simulink model "sim_process_power_old"  (Simulink 9.3)
settings: Solver=VariableStepAuto  StartTime=0.0  StopTime=0.1  MaxStep=1/25e3  RelTol=1e-3
settings Model: Creator=VMORAIS  LastModifiedBy=VMORAIS
settings DataIOCC: SaveFormat=Dataset  SignalLoggingSaveFormat=Dataset  ReturnWorkspaceOutputs=on
settings OptimizationCC: LifeSpan=auto
settings DebuggingCC: UnderspecifiedInitializationDetection=Simplified  MergeDetectMultiDrivingBlocksExec=error  FcnCallInpInsideContextMsg=error  SFUnexpectedBacktrackingDiag=error  SFNoUnconditionalDefaultTransitionDiag=error  SFExecutionAtInitializationDiag=warning  SFMachineParentedDataDiag=error  ArithmeticOperatorsInVariantConditions=error
settings HardwareCC: ProdBitPerPointer=64  ProdBitPerSizeT=64  ProdBitPerPtrDiffT=64  ProdLargestAtomicFloat=Float  ProdIntDivRoundTo=Zero  ProdEndianess=LittleEndian  ProdWordSize=64  ProdHWDeviceType=Intel->x86-64 (Windows64)
settings ModelReferenceCC: PropagateSignalLabelsOutOfModel=on
settings SFSimCC: SimUseLocalCustomCode=on
settings RTWCC: RTWUseLocalCustomCode=on
settings CodeAppCC: StateflowObjectComments=off
settings GRTTargetCC: TargetLangStandard=C99 (ISO)  CombineOutputUpdateFcns=on  GRTInterface=off
settings ConfigComp: CovMetricSettings=dwe  CovSaveCumulativeToWorkspaceVar=off  CovSaveSingleToWorkspaceVar=off  CovExternalEMLEnable=on

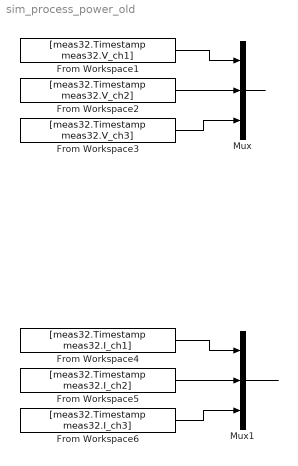
== system sim_process_power_old ==
  From Workspace1 : FromWorkspace  VariableName=[meas32.Timestamp meas32.V_ch1]  SampleTime=-1
  From Workspace2 : FromWorkspace  VariableName=[meas32.Timestamp meas32.V_ch2]  SampleTime=-1
  From Workspace3 : FromWorkspace  VariableName=[meas32.Timestamp meas32.V_ch3]  SampleTime=-1
  From Workspace4 : FromWorkspace  VariableName=[meas32.Timestamp meas32.I_ch1]  SampleTime=-1
  From Workspace5 : FromWorkspace  VariableName=[meas32.Timestamp meas32.I_ch2]  SampleTime=-1
  From Workspace6 : FromWorkspace  VariableName=[meas32.Timestamp meas32.I_ch3]  SampleTime=-1
  Mux : Mux  Inputs=3
  Mux1 : Mux  Inputs=3
  wires:
  From Workspace2/1 -> Mux/2
  From Workspace1/1 -> Mux/1
  From Workspace3/1 -> Mux/3
  Mux/1 -> ?
  From Workspace6/1 -> Mux1/3
  From Workspace4/1 -> Mux1/1
  From Workspace5/1 -> Mux1/2
  Mux1/1 -> ?
